simulink model "TFlex_ISSGPcopy"  (R2018b)
settings: Solver=VariableStepAuto  StartTime=0.0  StopTime=t_end  RelTol=1e-3
values from neighbouring files (symbols this model uses):
  b_init = ones(2*D,1).*0.0001    [TFlex_ISSGP_init.m]
  D = 80    [TFlex_ISSGP_Twin_init.m]    (also in TFlex_ISSGP_init.m = 21)
  n = 3    [TFlex_ISSGP_Twin_init.m]    (also in TFlex_ISSGP_init.m)
  R_init = eye(2*D,2*D).*sn    [TFlex_ISSGP_init.m]
  sf = 1    [TFlex_ISSGP_Twin_init.m]    (also in TFlex_ISSGP_init.m = 101.81)
  SIGMA = RAND.*(1./l)    [TFlex_ISSGP_init.m]
  sn = 2.303584    [TFlex_ISSGP_Twin_init.m]    (also in TFlex_ISSGP_init.m = 1.4493)
  t_learn = 55    [TFlex_ISSGP_Twin_init.m]    (also in TFlex_ISSGP_init.m = 1)
  t_predict = 65    [TFlex_ISSGP_Twin_init.m]    (also in TFlex_ISSGP_init.m = 41)
  ts = 1/1000    (= 0.001)    [TFlex_ISSGP_Twin_init.m]    (also in TFlex_ISSGP_init.m)
  w_init = ones(2*D,1)*sn    [TFlex_ISSGP_init.m]
undefined symbols (not defined in the file or in its folder): Cogging, DiscIntNeverNeededParam, gravity, Hysteresis, I_limit, PID, Plant, R1, R2, Reference, SVF
libraries: simulink x4
settings Model: Creator=wout7  LastModifiedBy=wout7

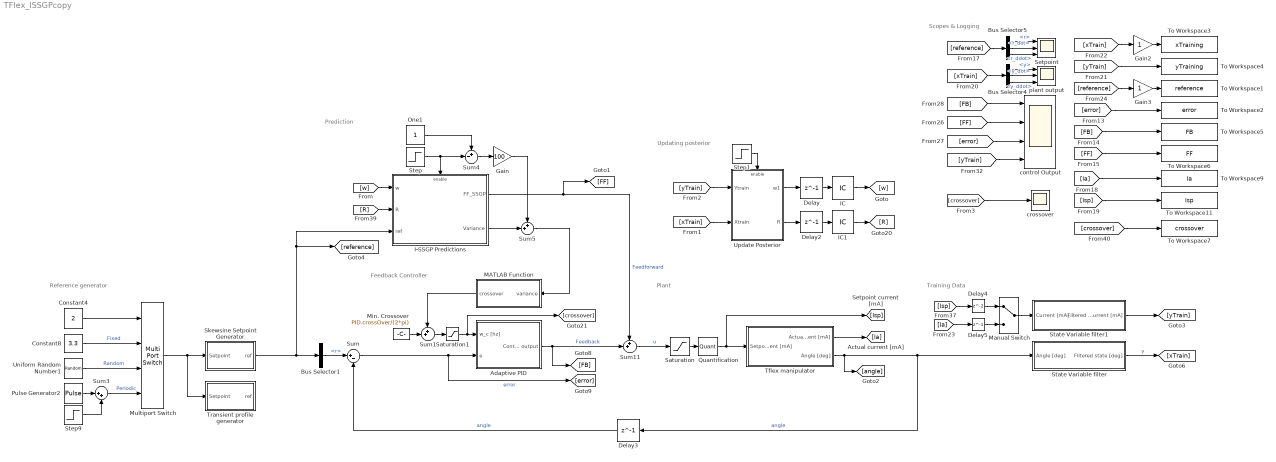
== system TFlex_ISSGPcopy ==
  note: Feedback Controller
  note: Training Data
  note: Plant
  note: Reference generator
  note: Scopes & Logging
  note: Updating posterior
  note: Prediction
  Adaptive PID : Subsystem
  Bus Selector1 : BusSelector  OutputSignals=r
  Bus Selector4 : BusSelector  OutputSignals=y,y_dot,y_ddot
  Bus Selector5 : BusSelector  OutputSignals=r,r_dot,r_ddot
  Constant4 : Constant  Value=2  SampleTime=Reference.ts
  Constant8 : Constant  Value=3.3  SampleTime=Reference.ts
  Delay : Delay  DelayLength=1  InitialCondition=0
  Delay2 : Delay  DelayLength=1  InitialCondition=0
  Delay3 : Delay  DelayLength=1  InitialCondition=0
  Delay4 : Delay
  Delay5 : Delay  DelayLength=1
  Gain : Gain  Gain=100
  Gain2 : Gain
  Gain3 : Gain
  I-SSGP Predictions : Subsystem
  IC : InitialCondition  Value=w_init
  IC1 : InitialCondition  Value=R_init
  MATLAB Function : MATLAB Function  TreatAsAtomicUnit=on
  Manual Switch : ManualSwitch
  Min. Crossover : Constant  Value=PID.crossOver/(2*pi)  OutDataTypeStr=Inherit: Inherit via back propagation
  Multiport Switch : MultiPortSwitch
  One1 : Constant  OutDataTypeStr=Inherit: Inherit via back propagation
  Pulse Generator2 : DiscretePulseGenerator  Amplitude=2*10  SampleTime=Reference.ts
  Quantification : Quantizer  QuantizationInterval=1
  Saturation : Saturate  UpperLimit=I_limit  LowerLimit=-I_limit
  Saturation1 : Saturate  UpperLimit=20  LowerLimit=0
  Setpoint : Scope  NumInputPorts=3
  Skewsine Setpoint Generator : Subsystem
  State Variable filter : Subsystem
  State Variable filter1 : Subsystem
  Step : Step  Time=t_predict  SampleTime=ts
  Step1 : Step  Time=t_learn  SampleTime=ts
  Step9 : Step  Time=0  After=-10  SampleTime=Reference.ts
  Sum : Sum  Inputs=|+-
  Sum1 : Sum  Inputs=++|
  Sum11 : Sum  Inputs=++|
  Sum3 : Sum  Inputs=|++
  Sum4 : Sum  Inputs=+-|
  Sum5 : Sum  Inputs=++|
  Tflex manipulator : Subsystem
  To Workspace1 : ToWorkspace  VariableName=reference  SampleTime=-1
  To Workspace11 : ToWorkspace  VariableName=Isp  SampleTime=-1
  To Workspace2 : ToWorkspace  VariableName=error  SampleTime=-1
  To Workspace3 : ToWorkspace  VariableName=xTraining  SampleTime=-1
  To Workspace4 : ToWorkspace  VariableName=yTraining  SampleTime=-1
  To Workspace5 : ToWorkspace  VariableName=FB  SampleTime=-1
  To Workspace6 : ToWorkspace  VariableName=FF  SampleTime=-1
  To Workspace7 : ToWorkspace  VariableName=crossover  SampleTime=-1
  To Workspace9 : ToWorkspace  VariableName=Ia  SampleTime=-1
  "Transient profile generator " : Subsystem
  Uniform Random Number1 : UniformRandomNumber  Minimum=-10  Maximum=10  Seed=Reference.seed  SampleTime=Reference.ts
  Update Posterior : Subsystem
  control Output : Scope  NumInputPorts=4
  crossover : Scope
  plant output : Scope  NumInputPorts=3
  wires:
  Bus Selector1/1 -> Sum/1  "<r>"
  Step/1 -> Sum4/2, I-SSGP Predictions/Enable
  IC/1 -> [w]
  [w] -> I-SSGP Predictions/1(w)
  Delay/1 -> IC/1
  [reference] -> Gain3/1
  Bus Selector5/2 -> Setpoint/2  "<r_dot>"
  Bus Selector5/1 -> Setpoint/1  "<r>"
  [error] -> To Workspace2/1
  Bus Selector5/3 -> Setpoint/3  "<r_ddot>"
  [FB] -> To Workspace5/1
  [xTrain] -> Gain2/1
  Gain2/1 -> To Workspace3/1
  [xTrain] -> Bus Selector4/1
  Gain3/1 -> To Workspace1/1
  Bus Selector4/1 -> plant output/1  "<y>"
  Bus Selector4/3 -> plant output/3  "<y_ddot>"
  [reference] -> Bus Selector5/1
  [yTrain] -> To Workspace4/1
  Bus Selector4/2 -> plant output/2  "<y_dot>"
  [FF] -> To Workspace6/1
  [yTrain] -> control Output/4
  [FF] -> control Output/2
  [error] -> control Output/3
  [FB] -> control Output/1
  Saturation/1 -> Quantification/1
  Adaptive PID/1(Control output) -> [FB], Sum11/2  "Feedback"
  Sum11/1 -> Saturation/1  "u"
  Quantification/1 -> [Isp], Tflex manipulator/1(Setpoint Current [mA])
  I-SSGP Predictions/1(FF_SSGP) -> Sum11/1, [FF]  "Feedforward"
  Pulse Generator2/1 -> Sum3/1
  Sum3/1 -> Multiport Switch/4  "Periodic"
  Step9/1 -> Sum3/2
  Constant4/1 -> Multiport Switch/1
  Uniform Random Number1/1 -> Multiport Switch/3  "Random"
  Constant8/1 -> Multiport Switch/2  "Fixed"
  [Ia] -> To Workspace9/1
  [Isp] -> To Workspace11/1
  State Variable filter1/1(Filtered Current [mA]) -> [yTrain]
  Skewsine Setpoint Generator/1(ref) -> Bus Selector1/1, I-SSGP Predictions/3(ref), [reference]
  Multiport Switch/1 -> "Transient profile generator "/1(Setpoint), Skewsine Setpoint Generator/1(Setpoint)
  Step1/1 -> Update Posterior/Enable
  [yTrain] -> Update Posterior/1(Ytrain)
  [xTrain] -> Update Posterior/2(Xtrain)
  Update Posterior/1(w1) -> Delay/1
  Delay2/1 -> IC1/1
  IC1/1 -> [R]
  Update Posterior/2(R) -> Delay2/1
  [R] -> I-SSGP Predictions/2(R)
  Min. Crossover/1 -> Sum1/2
  Saturation1/1 -> [crossover], Adaptive PID/1(w_c [hz])
  Sum1/1 -> Saturation1/1
  [crossover] -> To Workspace7/1
  Sum5/1 -> MATLAB Function/1(variance)
  [Isp] -> Delay4/1
  State Variable filter/1(Filtered state [deg]) -> [xTrain]  "y"
  [Ia] -> Delay5/1
  Delay4/1 -> Manual Switch/1
  Delay3/1 -> Sum/2  "angle"
  One1/1 -> Sum4/1
  I-SSGP Predictions/2(Variance) -> Sum5/2
  Sum4/1 -> Gain/1
  Gain/1 -> Sum5/1
  Tflex manipulator/2(Angle [deg]) -> Delay3/1, State Variable filter/1(Angle [deg]), [angle]  "angle"
  Tflex manipulator/1(Actual Current [mA]) -> [Ia]
  Delay5/1 -> Manual Switch/2
  Manual Switch/1 -> State Variable filter1/1(Current [mA])
  Sum/1 -> [error], Adaptive PID/2(e)  "error"
  MATLAB Function/1(crossover) -> Sum1/1
  [crossover] -> crossover/1

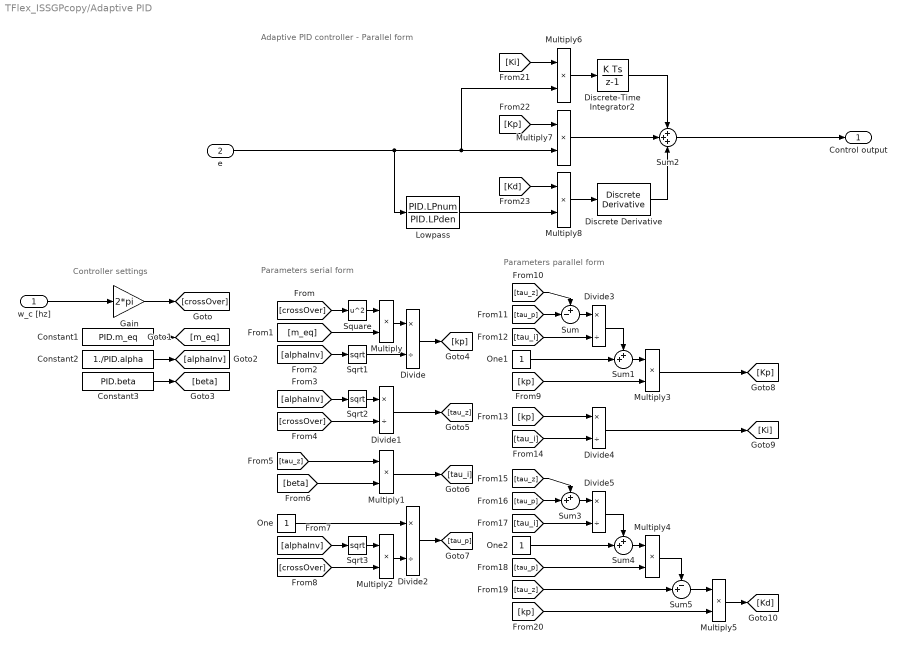
== system TFlex_ISSGPcopy/Adaptive PID ==
  note: Adaptive PID controller - Parallel form
  note: Controller settings
  note: Parameters parallel form
  note: Parameters serial form
  w_c [hz] : Inport
  e : Inport  Port=2
  Constant1 : Constant  Value=PID.m_eq
  Constant2 : Constant  Value=1./PID.alpha
  Constant3 : Constant  Value=PID.beta
  Discrete Derivative : simulink/Discrete/Discrete Derivative  gainval=1.0  ICPrevScaledInput=0.0  OutMin=[]  OutMax=[]  OutDataType=fixdt(1, 16)  OutScaling=2^-10  DoSatur=off
  Discrete-Time Integrator2 : DiscreteIntegrator  SampleTime=-1  ICPrevOutput=DiscIntNeverNeededParam  ICPrevScaledInput=DiscIntNeverNeededParam
  Divide{,1..5} (6 alike) : Product  Inputs=*/
  Gain : Gain  Gain=2*pi
  Lowpass : DiscreteTransferFcn  Numerator=PID.LPnum  Denominator=PID.LPden  SampleTime=ts
  Multiply{,1..8} (9 alike) : Product
  One : Constant  OutDataTypeStr=Inherit: Inherit via back propagation
  One1 : Constant  OutDataTypeStr=Inherit: Inherit via back propagation
  One2 : Constant  OutDataTypeStr=Inherit: Inherit via back propagation
  Sqrt1 : Sqrt  SaturateOnIntegerOverflow=on
  Sqrt2 : Sqrt  SaturateOnIntegerOverflow=on
  Sqrt3 : Sqrt  SaturateOnIntegerOverflow=on
  Square : Math  Operator=square  SaturateOnIntegerOverflow=on
  Sum : Sum  Inputs=+-|
  Sum1 : Sum  Inputs=++|
  Sum2 : Sum  Inputs=3
  Sum3 : Sum  Inputs=++|
  Sum4 : Sum  Inputs=++|
  Sum5 : Sum  Inputs=-+|
  Control output : Outport
  wires:
  w_c [hz]/1 -> Gain/1
  Constant1/1 -> [m_eq]
  Constant2/1 -> [alphaInv]
  Constant3/1 -> [beta]
  [crossOver] -> Square/1
  Square/1 -> Multiply/1
  [m_eq] -> Multiply/2
  [alphaInv] -> Sqrt1/1
  Multiply/1 -> Divide/1
  Sqrt1/1 -> Divide/2
  Divide/1 -> [kp]
  [alphaInv] -> Sqrt2/1
  Sqrt2/1 -> Divide1/1
  [crossOver] -> Divide1/2
  Divide1/1 -> [tau_z]
  [tau_z] -> Multiply1/1
  [beta] -> Multiply1/2
  Multiply1/1 -> [tau_i]
  Sqrt3/1 -> Multiply2/1
  [crossOver] -> Multiply2/2
  [alphaInv] -> Sqrt3/1
  One/1 -> Divide2/1
  Multiply2/1 -> Divide2/2
  Divide2/1 -> [tau_p]
  [tau_z] -> Sum/1
  [tau_p] -> Sum/2
  Sum/1 -> Divide3/1
  [tau_i] -> Divide3/2
  Divide3/1 -> Sum1/1
  One1/1 -> Sum1/2
  Sum1/1 -> Multiply3/1
  [kp] -> Multiply3/2
  Multiply3/1 -> [Kp]
  [kp] -> Divide4/1
  [tau_i] -> Divide4/2
  Divide4/1 -> [Ki]
  [tau_i] -> Divide5/2
  Sum3/1 -> Divide5/1
  [tau_z] -> Sum3/1
  [tau_p] -> Sum3/2
  Divide5/1 -> Sum4/1
  One2/1 -> Sum4/2
  Sum4/1 -> Multiply4/1
  [tau_p] -> Multiply4/2
  Multiply4/1 -> Sum5/1
  [tau_z] -> Sum5/2
  Sum5/1 -> Multiply5/1
  [kp] -> Multiply5/2
  Multiply5/1 -> [Kd]
  Multiply6/1 -> Discrete-Time Integrator2/1
  Sum2/1 -> Control output/1
  e/1 -> Multiply6/2, Multiply7/2, Lowpass/1
  Multiply8/1 -> Discrete Derivative/1
  [Kd] -> Multiply8/1
  Lowpass/1 -> Multiply8/2
  [Kp] -> Multiply7/1
  [Ki] -> Multiply6/1
  Multiply7/1 -> Sum2/2
  Gain/1 -> [crossOver]
  Discrete-Time Integrator2/1 -> Sum2/1
  Discrete Derivative/1 -> Sum2/3

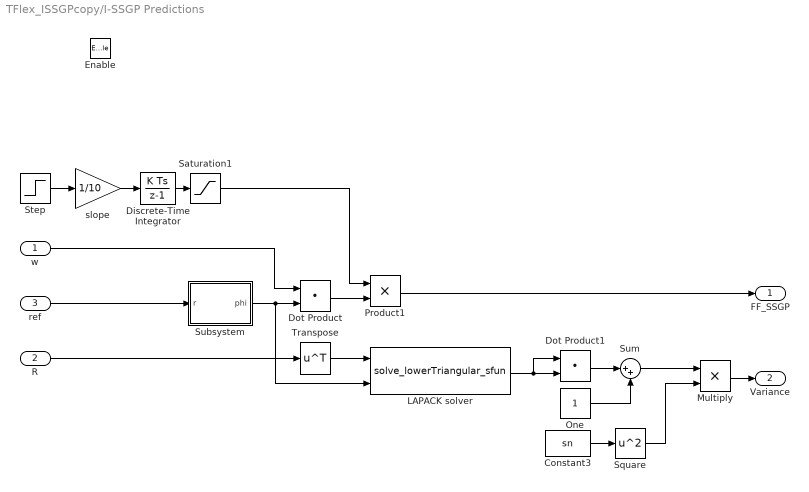
== system TFlex_ISSGPcopy/I-SSGP Predictions ==
  w : Inport
  R : Inport  Port=2
  ref : Inport  Port=3
  Enable : EnablePort
  Constant3 : Constant  Value=sn  SampleTime=-1
  Discrete-Time Integrator : DiscreteIntegrator  SampleTime=-1  ICPrevOutput=DiscIntNeverNeededParam  ICPrevScaledInput=DiscIntNeverNeededParam
  Dot Product : DotProduct  OutDataTypeStr=Inherit: Inherit via internal rule
  Dot Product1 : DotProduct  OutDataTypeStr=Inherit: Inherit via internal rule
  LAPACK solver : S-Function  FunctionName=solve_lowerTriangular_sfun  Parameters=2*D  SFunctionDeploymentMode=off  EnableBusSupport=off
  Multiply : Product
  One : Constant  OutDataTypeStr=Inherit: Inherit via back propagation
  Product1 : Product
  Saturation1 : Saturate  UpperLimit=1  LowerLimit=0
  Square : Math  Operator=square  SaturateOnIntegerOverflow=on
  Step : Step  Time=t_predict  SampleTime=ts
  Subsystem : Subsystem
  Sum : Sum  Inputs=|++
  Transpose : Math  Operator=transpose  SaturateOnIntegerOverflow=on
  slope : Gain  Gain=1/10
  FF_SSGP : Outport  SampleTime=ts
  Variance : Outport  Port=2  SampleTime=ts
  wires:
  w/1 -> Dot Product/1
  Subsystem/1(phi) -> LAPACK solver/2, Dot Product/2
  Product1/1 -> FF_SSGP/1
  Dot Product/1 -> Product1/2
  Saturation1/1 -> Product1/1
  ref/1 -> Subsystem/1(r)
  R/1 -> Transpose/1
  Transpose/1 -> LAPACK solver/1
  LAPACK solver/1 -> Dot Product1/1, Dot Product1/2
  Constant3/1 -> Square/1
  Multiply/1 -> Variance/1
  Dot Product1/1 -> Sum/1
  Sum/1 -> Multiply/1
  One/1 -> Sum/2
  Square/1 -> Multiply/2
  slope/1 -> Discrete-Time Integrator/1
  Discrete-Time Integrator/1 -> Saturation1/1
  Step/1 -> slope/1

== system TFlex_ISSGPcopy/Skewsine Setpoint Generator ==
  Setpoint : Inport
  Bus Creator : BusCreator  Inputs=3
  Subsystem : Subsystem
  ref : Outport
  wires:
  Subsystem/3(r_ddot) -> Bus Creator/3  "r_ddot"
  Bus Creator/1 -> ref/1
  Subsystem/2(r_dot) -> Bus Creator/2  "r_dot"
  Subsystem/1(r) -> Bus Creator/1  "r"
  Setpoint/1 -> Subsystem/1(setpoint)

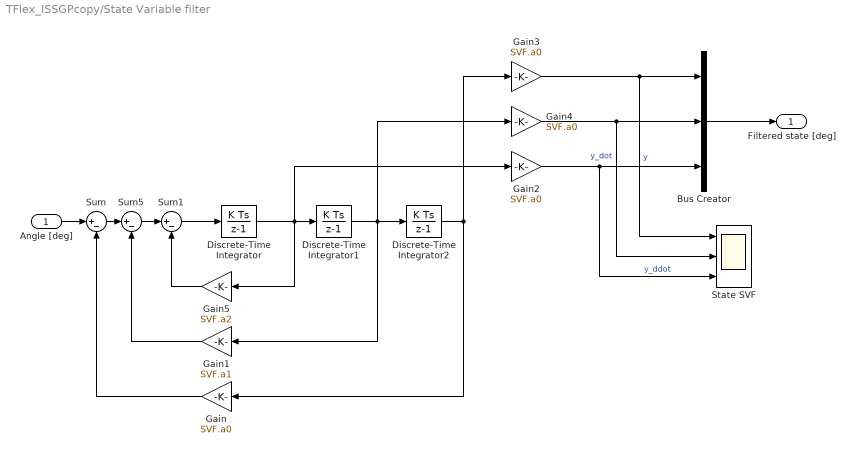
== system TFlex_ISSGPcopy/State Variable filter ==
  Angle [deg] : Inport
  Bus Creator : BusCreator  Inputs=3
  Discrete-Time Integrator : DiscreteIntegrator  SampleTime=-1  ICPrevOutput=DiscIntNeverNeededParam  ICPrevScaledInput=DiscIntNeverNeededParam
  Discrete-Time Integrator1 : DiscreteIntegrator  SampleTime=-1  ICPrevOutput=DiscIntNeverNeededParam  ICPrevScaledInput=DiscIntNeverNeededParam
  Discrete-Time Integrator2 : DiscreteIntegrator  SampleTime=-1  ICPrevOutput=DiscIntNeverNeededParam  ICPrevScaledInput=DiscIntNeverNeededParam
  Gain{,2..4} (4 alike) : Gain  Gain=SVF.a0
  Gain1 : Gain  Gain=SVF.a1
  Gain5 : Gain  Gain=SVF.a2
  State SVF : Scope  NumInputPorts=3
  Sum : Sum  Inputs=|+-
  Sum1 : Sum  Inputs=|+-
  Sum5 : Sum  Inputs=|+-
  Filtered state [deg] : Outport  SampleTime=ts
  wires:
  Bus Creator/1 -> Filtered state [deg]/1
  Sum1/1 -> Discrete-Time Integrator/1
  Angle [deg]/1 -> Sum/1
  Sum/1 -> Sum5/1
  Gain/1 -> Sum/2
  Gain1/1 -> Sum5/2
  Gain3/1 -> State SVF/1, Bus Creator/1  "y"
  Gain2/1 -> State SVF/3, Bus Creator/3  "y_ddot"
  Gain4/1 -> State SVF/2, Bus Creator/2  "y_dot"
  Gain5/1 -> Sum1/2
  Sum5/1 -> Sum1/1
  Discrete-Time Integrator/1 -> Discrete-Time Integrator1/1, Gain2/1, Gain5/1
  Discrete-Time Integrator1/1 -> Discrete-Time Integrator2/1, Gain4/1, Gain1/1
  Discrete-Time Integrator2/1 -> Gain3/1, Gain/1

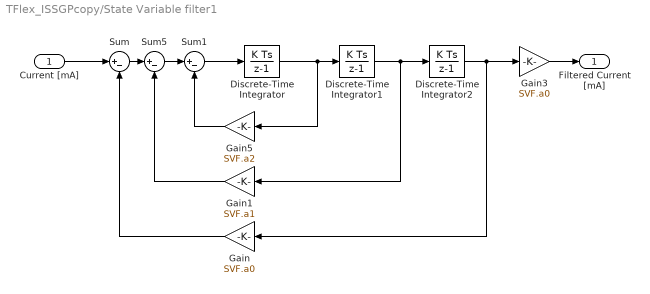
== system TFlex_ISSGPcopy/State Variable filter1 ==
  Current [mA] : Inport
  Discrete-Time Integrator : DiscreteIntegrator  SampleTime=-1  ICPrevOutput=DiscIntNeverNeededParam  ICPrevScaledInput=DiscIntNeverNeededParam
  Discrete-Time Integrator1 : DiscreteIntegrator  SampleTime=-1  ICPrevOutput=DiscIntNeverNeededParam  ICPrevScaledInput=DiscIntNeverNeededParam
  Discrete-Time Integrator2 : DiscreteIntegrator  SampleTime=-1  ICPrevOutput=DiscIntNeverNeededParam  ICPrevScaledInput=DiscIntNeverNeededParam
  Gain : Gain  Gain=SVF.a0
  Gain1 : Gain  Gain=SVF.a1
  Gain3 : Gain  Gain=SVF.a0
  Gain5 : Gain  Gain=SVF.a2
  Sum : Sum  Inputs=|+-
  Sum1 : Sum  Inputs=|+-
  Sum5 : Sum  Inputs=|+-
  Filtered Current [mA] : Outport  SampleTime=ts
  wires:
  Sum1/1 -> Discrete-Time Integrator/1
  Current [mA]/1 -> Sum/1
  Sum/1 -> Sum5/1
  Gain/1 -> Sum/2
  Gain1/1 -> Sum5/2
  Gain3/1 -> Filtered Current [mA]/1
  Gain5/1 -> Sum1/2
  Sum5/1 -> Sum1/1
  Discrete-Time Integrator/1 -> Discrete-Time Integrator1/1, Gain5/1
  Discrete-Time Integrator1/1 -> Discrete-Time Integrator2/1, Gain1/1
  Discrete-Time Integrator2/1 -> Gain3/1, Gain/1

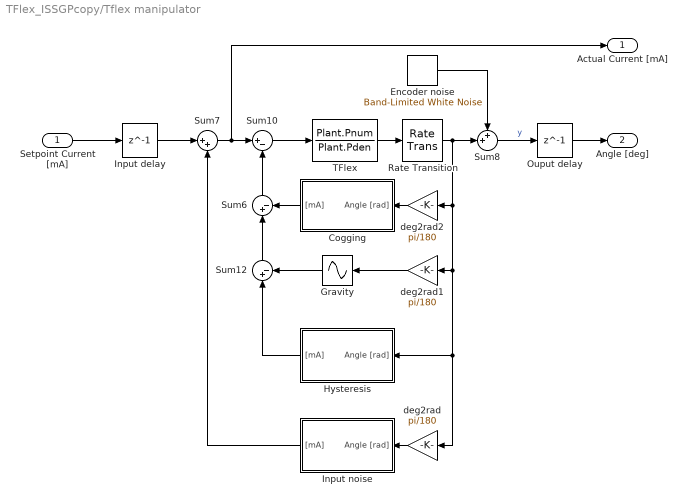
== system TFlex_ISSGPcopy/Tflex manipulator ==
  Setpoint Current [mA] : Inport
  Cogging : Subsystem
  Encoder noise : simulink/Sources/Band-Limited White Noise  Cov=[1e-13]  Ts=ts  seed=[23341]
  Gravity : Sin  TimeSource=Use external signal  Amplitude=gravity.constant  Phase=gravity.phase  SampleTime=0
  Hysteresis : Subsystem
  Input delay : Delay  DelayLength=1  InitialCondition=0
  Input noise : Subsystem
  Ouput delay : Delay  DelayLength=1  InitialCondition=0
  Rate Transition : RateTransition  OutPortSampleTime=ts
  Sum10 : Sum  Inputs=|+-
  Sum12 : Sum  Inputs=|+-
  Sum6 : Sum  Inputs=|+-
  Sum7 : Sum  Inputs=|++
  Sum8 : Sum  Inputs=++|
  TFlex : TransferFcn  Numerator=Plant.Pnum  Denominator=Plant.Pden  ContinuousStateAttributes='angle'
  deg2rad : Gain  Gain=pi/180
  deg2rad1 : Gain  Gain=pi/180
  deg2rad2 : Gain  Gain=pi/180
  Actual Current [mA] : Outport
  Angle [deg] : Outport  Port=2
  wires:
  Sum8/1 -> Ouput delay/1  "y"
  Rate Transition/1 -> Sum8/2, deg2rad2/1, deg2rad1/1, deg2rad/1, Hysteresis/1(Angle [rad])
  Sum7/1 -> Actual Current [mA]/1, Sum10/1
  Hysteresis/1("[mA]") -> Sum12/1
  TFlex/1 -> Rate Transition/1
  Cogging/1("[mA]") -> Sum6/2
  Gravity/1 -> Sum12/2
  Setpoint Current [mA]/1 -> Input delay/1
  Sum12/1 -> Sum6/1
  Ouput delay/1 -> Angle [deg]/1
  Sum10/1 -> TFlex/1
  Input delay/1 -> Sum7/1
  Sum6/1 -> Sum10/2
  Encoder noise/1 -> Sum8/1
  deg2rad1/1 -> Gravity/1
  Input noise/1("[mA]") -> Sum7/2
  deg2rad/1 -> Input noise/1(Angle [rad])
  deg2rad2/1 -> Cogging/1(Angle [rad])

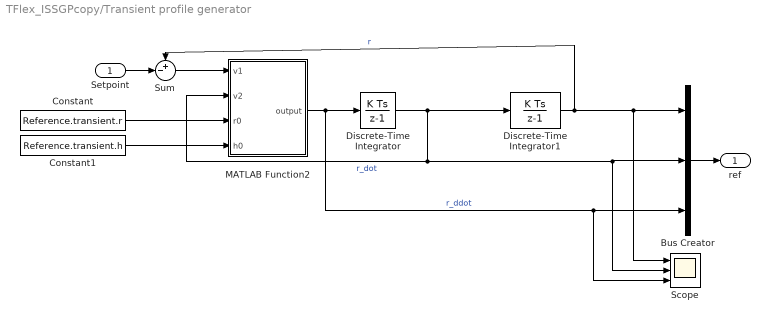
== system TFlex_ISSGPcopy/Transient profile generator  ==
  Setpoint : Inport
  Bus Creator : BusCreator  Inputs=3
  Constant : Constant  Value=Reference.transient.r  SampleTime=ts
  Constant1 : Constant  Value=Reference.transient.h  SampleTime=ts
  Discrete-Time Integrator : DiscreteIntegrator  gainval=1  SampleTime=ts  ICPrevOutput=DiscIntNeverNeededParam  ICPrevScaledInput=DiscIntNeverNeededParam
  Discrete-Time Integrator1 : DiscreteIntegrator  gainval=1  InitialCondition=-24  SampleTime=ts  ICPrevOutput=DiscIntNeverNeededParam  ICPrevScaledInput=DiscIntNeverNeededParam
  MATLAB Function2 : MATLAB Function  TreatAsAtomicUnit=on
  Scope : Scope  NumInputPorts=3
  Sum : Sum  Inputs=+-|
  ref : Outport
  wires:
  Sum/1 -> MATLAB Function2/1(v1)
  Setpoint/1 -> Sum/2
  Constant/1 -> MATLAB Function2/3(r0)
  Constant1/1 -> MATLAB Function2/4(h0)
  Discrete-Time Integrator1/1 -> Scope/1, Bus Creator/1, Sum/1  "r"
  Discrete-Time Integrator/1 -> Discrete-Time Integrator1/1, MATLAB Function2/2(v2), Bus Creator/2, Scope/2  "r_dot"
  Bus Creator/1 -> ref/1
  MATLAB Function2/1(output) -> Scope/3, Bus Creator/3, Discrete-Time Integrator/1  "r_ddot"

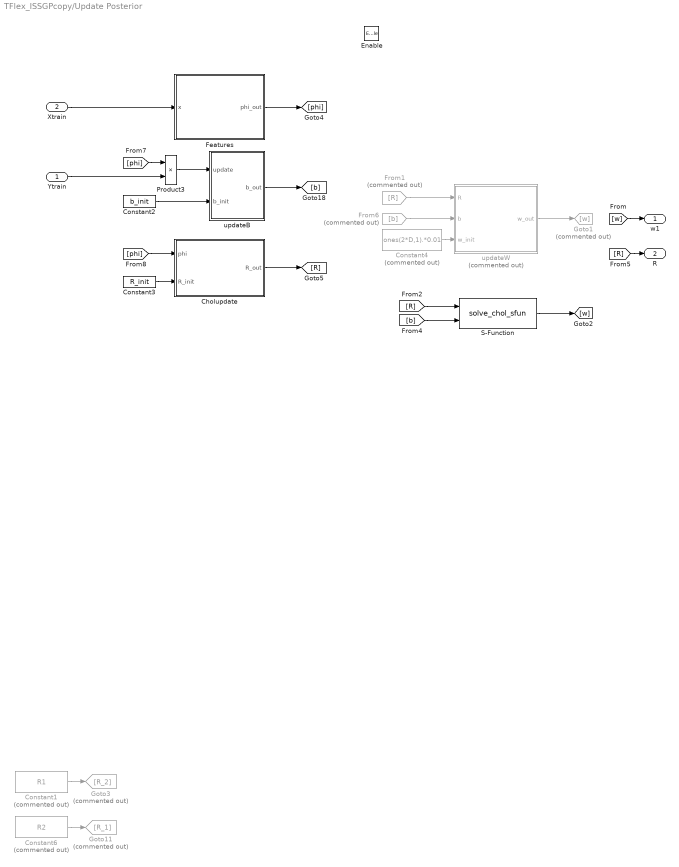
== system TFlex_ISSGPcopy/Update Posterior ==
  Ytrain : Inport  PortDimensions=[1,1]
  Xtrain : Inport  Port=2  PortDimensions=[n,1]
  Enable : EnablePort
  Cholupdate : MATLAB Function  TreatAsAtomicUnit=on
  Constant1 : Constant  Commented=on  Value=R1  VectorParams1D=off  SampleTime=-1
  Constant2 : Constant  Value=b_init  SampleTime=-1
  Constant3 : Constant  Value=R_init  SampleTime=-1
  Constant4 : Constant  Commented=on  Value=ones(2*D,1).*0.01  SampleTime=ts
  Constant6 : Constant  Commented=on  Value=R2  VectorParams1D=off  SampleTime=-1
  Features : Subsystem
  From1 : From  Commented=on  GotoTag=R
  From6 : From  Commented=on  GotoTag=b
  Goto1 : Goto  Commented=on  GotoTag=w
  Goto11 : Goto  Commented=on  GotoTag=R_1
  Goto3 : Goto  Commented=on  GotoTag=R_2
  Product3 : Product
  S-Function : S-Function  FunctionName=solve_chol_sfun  Parameters=2*D  SFunctionDeploymentMode=off  EnableBusSupport=off
  updateB : MATLAB Function  TreatAsAtomicUnit=on
  updateW : MATLAB Function  Commented=on  TreatAsAtomicUnit=on
  w1 : Outport
  R : Outport  Port=2
  wires:
  [phi] -> Cholupdate/1(phi)
  Features/1(phi_out) -> [phi]
  Cholupdate/1(R_out) -> [R]
  From1/1 -> updateW/1(R)
  From6/1 -> updateW/2(b)
  Constant1/1 -> Goto3/1
  Constant6/1 -> Goto11/1
  Ytrain/1 -> Product3/2
  [phi] -> Product3/1
  Product3/1 -> updateB/1(update)
  updateB/1(b_out) -> [b]
  Xtrain/1 -> Features/1(x)
  Constant3/1 -> Cholupdate/2(R_init)
  Constant2/1 -> updateB/2(b_init)
  Constant4/1 -> updateW/3(w_init)
  [R] -> S-Function/1
  [b] -> S-Function/2
  [w] -> w1/1
  updateW/1(w_out) -> Goto1/1
  S-Function/1 -> [w]
  [R] -> R/1

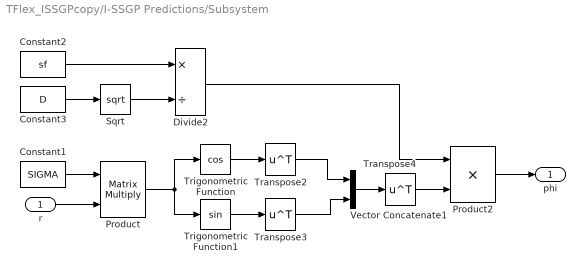
== system TFlex_ISSGPcopy/I-SSGP Predictions/Subsystem ==
  r : Inport
  Constant1 : Constant  Value=SIGMA  SampleTime=-1
  Constant2 : Constant  Value=sf  SampleTime=-1
  Constant3 : Constant  Value=D  SampleTime=-1
  Divide2 : Product  Inputs=*/
  Product : Product  Multiplication=Matrix(*)
  Product2 : Product
  Sqrt : Sqrt  SaturateOnIntegerOverflow=on
  Transpose2 : Math  Operator=transpose  SaturateOnIntegerOverflow=on
  Transpose3 : Math  Operator=transpose  SaturateOnIntegerOverflow=on
  Transpose4 : Math  Operator=transpose  SaturateOnIntegerOverflow=on
  Trigonometric Function : Trigonometry  Operator=cos
  Trigonometric Function1 : Trigonometry
  Vector Concatenate1 : Concatenate
  phi : Outport
  wires:
  r/1 -> Product/2
  Product/1 -> Trigonometric Function1/1, Trigonometric Function/1
  Product2/1 -> phi/1
  Constant2/1 -> Divide2/1
  Divide2/1 -> Product2/1
  Transpose2/1 -> Vector Concatenate1/1
  Transpose4/1 -> Product2/2
  Constant3/1 -> Sqrt/1
  Trigonometric Function1/1 -> Transpose3/1
  Trigonometric Function/1 -> Transpose2/1
  Vector Concatenate1/1 -> Transpose4/1
  Transpose3/1 -> Vector Concatenate1/2
  Sqrt/1 -> Divide2/2
  Constant1/1 -> Product/1

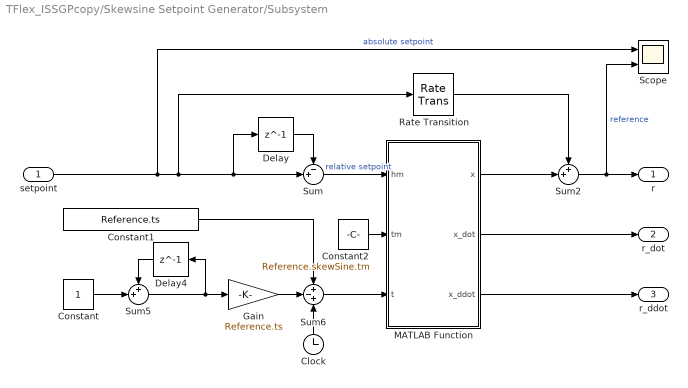
== system TFlex_ISSGPcopy/Skewsine Setpoint Generator/Subsystem ==
  setpoint : Inport
  Clock : Clock
      settings: Decimation=100
  Constant : Constant  SampleTime=Reference.ts
  Constant1 : Constant  Value=Reference.ts  SampleTime=Reference.ts
  Constant2 : Constant  Value=Reference.skewSine.tm  SampleTime=Reference.ts
  Delay : Delay  DelayLength=1  InitialCondition=0  SampleTime=Reference.ts
  Delay4 : Delay  DelayLength=1  InitialCondition=0  SampleTime=Reference.ts
  Gain : Gain  Gain=Reference.ts
  MATLAB Function : MATLAB Function  TreatAsAtomicUnit=on
  Rate Transition : RateTransition  OutPortSampleTime=ts
  Scope : Scope  NumInputPorts=2
  Sum : Sum  Inputs=-+|
  Sum2 : Sum  Inputs=++|
  Sum5 : Sum  Inputs=++|
  Sum6 : Sum  Inputs=+-+
  r : Outport
  r_dot : Outport  Port=2
  r_ddot : Outport  Port=3
  wires:
  Delay4/1 -> Sum5/1
  Sum2/1 -> r/1, Scope/2  "reference"
  Sum5/1 -> Delay4/1, Gain/1
  Constant/1 -> Sum5/2
  MATLAB Function/3(x_ddot) -> r_ddot/1
  Clock/1 -> Sum6/3
  Delay/1 -> Sum/1
  Gain/1 -> Sum6/2
  Constant1/1 -> Sum6/1
  MATLAB Function/2(x_dot) -> r_dot/1
  Sum/1 -> MATLAB Function/1(hm)  "relative setpoint"
  Constant2/1 -> MATLAB Function/2(tm)
  Sum6/1 -> MATLAB Function/3(t)
  MATLAB Function/1(x) -> Sum2/2
  setpoint/1 -> Scope/1, Rate Transition/1, Delay/1, Sum/2  "absolute setpoint"
  Rate Transition/1 -> Sum2/1

== system TFlex_ISSGPcopy/Tflex manipulator/Cogging ==
  Angle [rad] : Inport
  Sine Wave Function : Sin  TimeSource=Use external signal  Amplitude=Cogging.amplitude  Frequency=Cogging.frequency*pi  Phase=Cogging.phase  SampleTime=0
  Sum of Elements : Sum  Inputs=+
  "[mA]" : Outport
  wires:
  Sum of Elements/1 -> "[mA]"/1
  Sine Wave Function/1 -> Sum of Elements/1
  Angle [rad]/1 -> Sine Wave Function/1

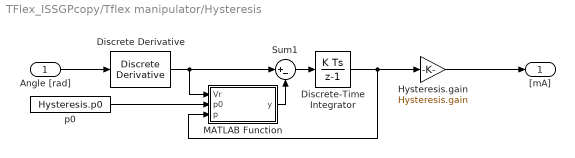
== system TFlex_ISSGPcopy/Tflex manipulator/Hysteresis ==
  Angle [rad] : Inport
  Discrete Derivative : simulink/Discrete/Discrete Derivative  gainval=1.0  ICPrevScaledInput=0.0  OutMin=[]  OutMax=[]  OutDataType=fixdt(1, 16)  OutScaling=2^-10  DoSatur=off
  Discrete-Time Integrator : DiscreteIntegrator  SampleTime=-1  ICPrevOutput=DiscIntNeverNeededParam  ICPrevScaledInput=DiscIntNeverNeededParam
  Hysteresis.gain : Gain  Gain=Hysteresis.gain
  MATLAB Function : MATLAB Function  TreatAsAtomicUnit=on
  Sum1 : Sum  Inputs=|+-
  p0 : Constant  Value=Hysteresis.p0
  "[mA]" : Outport
  wires:
  MATLAB Function/1(y) -> Sum1/2
  Angle [rad]/1 -> Discrete Derivative/1
  Sum1/1 -> Discrete-Time Integrator/1
  Discrete Derivative/1 -> Sum1/1, MATLAB Function/1(Vr)
  Discrete-Time Integrator/1 -> MATLAB Function/3(p), Hysteresis.gain/1
  Hysteresis.gain/1 -> "[mA]"/1
  p0/1 -> MATLAB Function/2(p0)

== system TFlex_ISSGPcopy/Tflex manipulator/Input noise ==
  Angle [rad] : Inport
  Band-Limited White Noise : simulink/Sources/Band-Limited White Noise  Cov=[1e-3]  Ts=ts  seed=48124
  Multiply2 : Product
  Noise variance : Sin  TimeSource=Use external signal  Bias=2  Frequency=27.7  SampleTime=0
  "[mA]" : Outport
  wires:
  Noise variance/1 -> Multiply2/2
  Angle [rad]/1 -> Noise variance/1
  Band-Limited White Noise/1 -> Multiply2/1
  Multiply2/1 -> "[mA]"/1

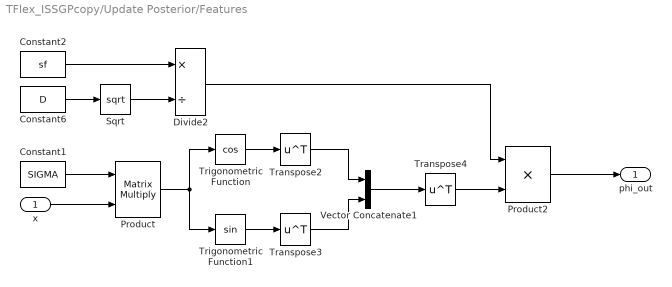
== system TFlex_ISSGPcopy/Update Posterior/Features ==
  x : Inport
  Constant1 : Constant  Value=SIGMA  SampleTime=-1
  Constant2 : Constant  Value=sf  SampleTime=-1
  Constant6 : Constant  Value=D  SampleTime=-1
  Divide2 : Product  Inputs=*/
  Product : Product  Multiplication=Matrix(*)
  Product2 : Product
  Sqrt : Sqrt  SaturateOnIntegerOverflow=on
  Transpose2 : Math  Operator=transpose  SaturateOnIntegerOverflow=on
  Transpose3 : Math  Operator=transpose  SaturateOnIntegerOverflow=on
  Transpose4 : Math  Operator=transpose  SaturateOnIntegerOverflow=on
  Trigonometric Function : Trigonometry  Operator=cos
  Trigonometric Function1 : Trigonometry
  Vector Concatenate1 : Concatenate
  phi_out : Outport
  wires:
  Constant1/1 -> Product/1
  Product2/1 -> phi_out/1
  Constant6/1 -> Sqrt/1
  Trigonometric Function1/1 -> Transpose3/1
  Trigonometric Function/1 -> Transpose2/1
  Vector Concatenate1/1 -> Transpose4/1
  Transpose3/1 -> Vector Concatenate1/2
  Product/1 -> Trigonometric Function1/1, Trigonometric Function/1
  x/1 -> Product/2
  Divide2/1 -> Product2/1
  Transpose4/1 -> Product2/2
  Sqrt/1 -> Divide2/2
  Transpose2/1 -> Vector Concatenate1/1
  Constant2/1 -> Divide2/1

== matlab function TFlex_ISSGPcopy/Skewsine Setpoint Generator/Subsystem/MATLAB Function ==
  settings: updateMethod=DISCRETE  sampleTime=ts
  data: hm input; x output; tm input; t input; x_dot output; x_ddot output
function [x,x_dot,x_ddot] = skewSine(hm,tm,t)

if (t>=0) && (t<=tm)
    x      = hm/tm*t - hm/(2*pi)*sin(2*pi/tm*t);
    x_dot  = hm/tm - hm/tm*cos(2*pi/tm*t);
    x_ddot = 2*pi*hm/(tm^2)*sin(2*pi/tm*t);
else
    x      = hm;
    x_dot  = 0;
    x_ddot = 0;
end

== matlab function TFlex_ISSGPcopy/Update Posterior/updateW ==
  settings: updateMethod=DISCRETE  sampleTime=ts
  data: R input size=[2*D,2*D]; w_out output size=[2*D,1]; b input; w_init input; D parameter
function w_out = updateW(R,b,w_init,D) 
persistent w
if(isempty(w))
    w = w_init;
end
coder.extrinsic('solve_chol');
w = solve_chol(R,b);
%w = R\(R'\b);
w_out = w;

== matlab function TFlex_ISSGPcopy/Tflex manipulator/Hysteresis/MATLAB Function ==
  data: Vr input; p0 input; y output; p input
function y = fcn(Vr,p0,p)
if Vr>0 && p>=p0
    y = Vr;
elseif Vr<0 && p<=-p0
    y = Vr;
else
    y = 0;
end

== matlab function TFlex_ISSGPcopy/Update Posterior/Cholupdate ==
  data: R_out output size=[2*D,2*D]; phi input; R_init input; D parameter; sn parameter
function R_out = cholupdate_fcn(phi, R_init, D, sn)
persistent R; 
if(isempty(R))
    R = R_init;
end
R = cholupdate(R,phi);
R_out = R;

== matlab function TFlex_ISSGPcopy/Transient profile generator /MATLAB Function2 ==
  data: v1 input; output output; v2 input; r0 input; h0 input
function output = Fhan(v1,v2,r0, h0)
d = h0^2*r0;
a0 = h0*v2;
y = v1 + a0;
a1 = sqrt(d*(d+8*abs(y)));
a2 = a0 + sign(y)*(a1-d)/2;
sy = (sign(y+d)-sign(y-d))/2;
a = (a0+y-a2)*sy +a2;
sa = (sign(a+d)-sign(a-d))/2;
output = -r0 *(a/d -sign(a) )*sa - r0*sign(a);

== matlab function TFlex_ISSGPcopy/Update Posterior/updateB ==
  settings: updateMethod=DISCRETE
  data: update input; b_init input; b_out output size=[2*D,1]; D parameter
function b_out = updateB(update, b_init, D)
persistent b 
if(isempty(b))
    b = b_init;
end

b = b + update;
b_out = b;

== matlab function TFlex_ISSGPcopy/MATLAB Function ==
  data: variance input; crossover output; sn parameter; PID parameter
function crossover  = variableCrossover(variance, sn, PID)
crossoverMax = 20;
crossoverMin = PID.crossOver/(2*pi);

z = (variance-sn.^2)*100;
z = min([z,1]);

crossover = z*(crossoverMax-crossoverMin);
